simulink model "LumpMassHeatXEx"  (R2015a)
settings: Solver=ode45  StartTime=0.0  StopTime=500  RelTol=1e-3
libraries: lib_GenHeatX_LumpedMassHeatX x2
settings Model: Creator=jlkratz  LastModifiedBy=jlkratz

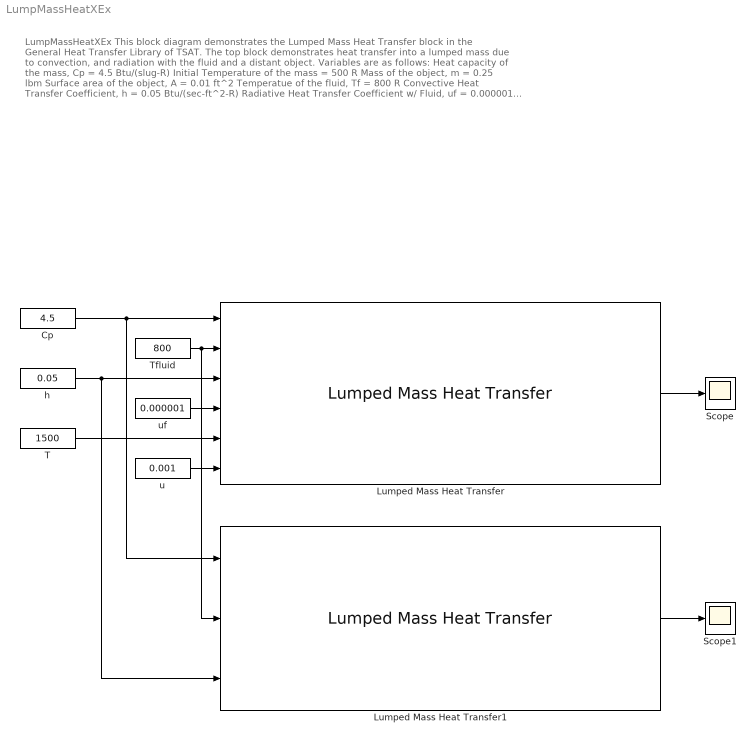
== system LumpMassHeatXEx ==
  note: LumpMassHeatXEx
      |
      | This block diagram demonstrates the Lumped Mass Heat Transfer block in the General Heat Transfer Library of TSAT. The top block
      | demonstrates heat transfer into a lumped mass due to convection, and radiation with the fluid and a distant object. Variables are as
      | follows:
      | Heat capacity of the mass, Cp = 4.5 Btu/(slug-R)
      | Initial Temperature of the mass = 500 R
      | Mass of the object, m = 0.25 lbm
      | Surface area of the object, A = 0.01 ft^2
      | Temperatue of the fluid, Tf = 800 R
      | Convective Heat Transfer Coefficient, h = 0.05 Btu/(sec-ft^2-R)
      | Radiative Heat Transfer Coefficient w/ Fluid, uf = 0.000001 Btu/(sec-ft^2-R)
      | Temperature of a distant object, Trad = 1500 R
      | Radiative Heat Transfer Coefficient w/ distant object = 0.001 Btu/(sec-ft^2-R)
      | The second instance of the block only consider heat transfer due to convection
  Cp : Constant  Value=4.5
  Lumped Mass Heat Transfer : lib_GenHeatX_LumpedMassHeatX/Lumped Mass Heat Transfer  Tmass0_M=500  m_M=0.25/32.174  conv_M=on  radf_M=on  Aconv_M=0.01  rads_M=on  Arad_M=0.01
  Lumped Mass Heat Transfer1 : lib_GenHeatX_LumpedMassHeatX/Lumped Mass Heat Transfer  Tmass0_M=500  m_M=0.25/32.174  conv_M=on  radf_M=off  Aconv_M=0.01  rads_M=off  Arad_M=0.01
  Scope : Scope
  Scope1 : Scope
  T : Constant  Value=1500
  Tfluid : Constant  Value=800
  h : Constant  Value=0.05
  u : Constant  Value=0.001
  uf : Constant  Value=0.000001
  wires:
  Tfluid/1 -> Lumped Mass Heat Transfer1/2, Lumped Mass Heat Transfer/2
  Cp/1 -> Lumped Mass Heat Transfer1/1, Lumped Mass Heat Transfer/1
  h/1 -> Lumped Mass Heat Transfer1/3, Lumped Mass Heat Transfer/3
  u/1 -> Lumped Mass Heat Transfer/6
  T/1 -> Lumped Mass Heat Transfer/5
  uf/1 -> Lumped Mass Heat Transfer/4
  Lumped Mass Heat Transfer/1 -> Scope/1
  Lumped Mass Heat Transfer1/1 -> Scope1/1
